simulink model "pid_model"  (R2017a)
settings: Solver=VariableStepAuto  StartTime=0.0  StopTime=10.0  RelTol=1e-3
values from neighbouring files (symbols this model uses):
  G_Denominator = str2double(get(hObject, 'String'))    [gui.m]    (also in variables.mat = [1 -4 3])
  G_Numerator = str2double(get(hObject, 'String'))    [gui.m]    (also in variables.mat = 1)
  H_Denominator = str2double(get(hObject, 'String'))    [gui.m]    (also in variables.mat = 1)
  H_Numerator = str2double(get(hObject, 'String'))    [gui.m]    (also in variables.mat = 1)
  phi_final = 10    [variables.mat]
  phi_initial = 0    [variables.mat]
  PID_D = str2double(get(hObject, 'String'))    [gui.m]    (also in variables.mat = 1000)
  PID_I = str2double(get(hObject, 'String'))    [gui.m]    (also in variables.mat = 0)
  PID_P = str2double(get(hObject, 'String'))    [gui.m]    (also in variables.mat = 17500)
  theta_final = 34    [variables.mat]
  theta_initial = 0    [variables.mat]
libraries: simulink x2
settings Model: Creator=arekmano  LastModifiedBy=arekmano

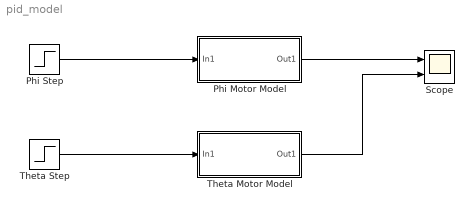
== system pid_model ==
  Phi Motor Model : Subsystem
  Phi Step : Step  Before=phi_initial  After=phi_final  SampleTime=0
  Scope : Scope  NumInputPorts=2
  Theta Motor Model : Subsystem
  Theta Step : Step  Before=theta_initial  After=theta_final  SampleTime=0
  wires:
  Phi Motor Model/1(Out1) -> Scope/1
  Phi Step/1 -> Phi Motor Model/1(In1)
  Theta Step/1 -> Theta Motor Model/1(In1)
  Theta Motor Model/1(Out1) -> Scope/2

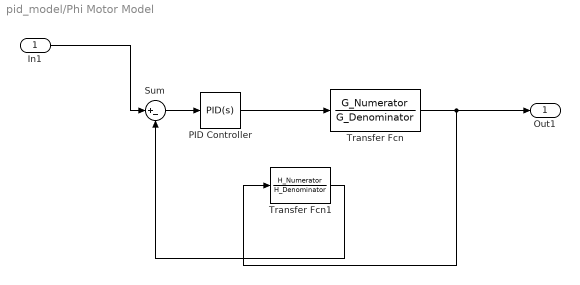
== system pid_model/Phi Motor Model ==
  In1 : Inport
  PID Controller : simulink/Continuous/PID Controller  Controller=PID  TimeDomain=Continuous-time  SampleTime=-1  IntegratorMethod=Forward Euler  FilterMethod=Forward Euler  Form=Parallel  UseFilter=on  ControllerParametersSource=internal  P=PID_P  I=PID_I  D=PID_D  N=6591903.7711168  InitialConditionSource=internal  InitialConditionForIntegrator=0  InitialConditionForFilter=0  ExternalReset=none  LimitOutput=off  UpperSaturationLimit=inf  LowerSaturationLimit=-inf  LinearizeAsGain=on  AntiWindupMode=none  Kb=1  TrackingMode=off  Kt=1  PParamMin=[]  PParamMax=[]  IParamMin=[]  IParamMax=[]  DParamMin=[]  DParamMax=[]  NParamMin=[]  NParamMax=[]  KbParamMin=[]  KbParamMax=[]  KtParamMin=[]  KtParamMax=[]  POutMin=[]  POutMax=[]  IOutMin=[]  IOutMax=[]  DOutMin=[]  DOutMax=[]  NOutMin=[]  NOutMax=[]  KbOutMin=[]  KbOutMax=[]  KtOutMin=[]  KtOutMax=[]  IntegratorOutMin=[]  IntegratorOutMax=[]  FilterOutMin=[]  FilterOutMax=[]  SumOutMin=[]  SumOutMax=[]  SumI1OutMin=[]  SumI1OutMax=[]  SumI2OutMin=[]  SumI2OutMax=[]  SumI3OutMin=[]  SumI3OutMax=[]  SumDOutMin=[]  SumDOutMax=[]  SaturationOutMin=[]  SaturationOutMax=[]  IntegratorContinuousStateAttributes=''  IntegratorStateMustResolveToSignalObject=off  IntegratorRTWStateStorageClass=Auto  FilterContinuousStateAttributes=''  FilterStateMustResolveToSignalObject=off  FilterRTWStateStorageClass=Auto  DifferentiatorICPrevScaledInput=0  DifferentiatorOutMin=[]  DifferentiatorOutMax=[]  InitialConditionSetting=State (most efficient)
  Sum : Sum  Inputs=|+-
  Transfer Fcn : TransferFcn  Numerator=G_Numerator  Denominator=G_Denominator
  Transfer Fcn1 : TransferFcn  Numerator=H_Numerator  Denominator=H_Denominator
  Out1 : Outport
  wires:
  In1/1 -> Sum/1
  PID Controller/1 -> Transfer Fcn/1
  Transfer Fcn/1 -> Transfer Fcn1/1, Out1/1
  Sum/1 -> PID Controller/1
  Transfer Fcn1/1 -> Sum/2

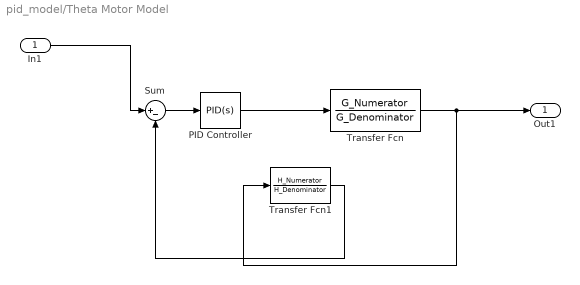
== system pid_model/Theta Motor Model ==
  In1 : Inport
  PID Controller : simulink/Continuous/PID Controller  Controller=PID  TimeDomain=Continuous-time  SampleTime=-1  IntegratorMethod=Forward Euler  FilterMethod=Forward Euler  Form=Parallel  UseFilter=on  ControllerParametersSource=internal  P=PID_P  I=PID_I  D=PID_D  N=6591903.7711168  InitialConditionSource=internal  InitialConditionForIntegrator=0  InitialConditionForFilter=0  ExternalReset=none  LimitOutput=off  UpperSaturationLimit=inf  LowerSaturationLimit=-inf  LinearizeAsGain=on  AntiWindupMode=none  Kb=1  TrackingMode=off  Kt=1  PParamMin=[]  PParamMax=[]  IParamMin=[]  IParamMax=[]  DParamMin=[]  DParamMax=[]  NParamMin=[]  NParamMax=[]  KbParamMin=[]  KbParamMax=[]  KtParamMin=[]  KtParamMax=[]  POutMin=[]  POutMax=[]  IOutMin=[]  IOutMax=[]  DOutMin=[]  DOutMax=[]  NOutMin=[]  NOutMax=[]  KbOutMin=[]  KbOutMax=[]  KtOutMin=[]  KtOutMax=[]  IntegratorOutMin=[]  IntegratorOutMax=[]  FilterOutMin=[]  FilterOutMax=[]  SumOutMin=[]  SumOutMax=[]  SumI1OutMin=[]  SumI1OutMax=[]  SumI2OutMin=[]  SumI2OutMax=[]  SumI3OutMin=[]  SumI3OutMax=[]  SumDOutMin=[]  SumDOutMax=[]  SaturationOutMin=[]  SaturationOutMax=[]  IntegratorContinuousStateAttributes=''  IntegratorStateMustResolveToSignalObject=off  IntegratorRTWStateStorageClass=Auto  FilterContinuousStateAttributes=''  FilterStateMustResolveToSignalObject=off  FilterRTWStateStorageClass=Auto  DifferentiatorICPrevScaledInput=0  DifferentiatorOutMin=[]  DifferentiatorOutMax=[]  InitialConditionSetting=State (most efficient)
  Sum : Sum  Inputs=|+-
  Transfer Fcn : TransferFcn  Numerator=G_Numerator  Denominator=G_Denominator
  Transfer Fcn1 : TransferFcn  Numerator=H_Numerator  Denominator=H_Denominator
  Out1 : Outport
  wires:
  In1/1 -> Sum/1
  PID Controller/1 -> Transfer Fcn/1
  Transfer Fcn/1 -> Transfer Fcn1/1, Out1/1
  Sum/1 -> PID Controller/1
  Transfer Fcn1/1 -> Sum/2
